simulink model "simulink_02"  (R2023b)
settings: Solver=VariableStepAuto  StartTime=0.0  StopTime=10000  RelTol=1e-3
settings Model: Creator=HP  LastModifiedBy=HP

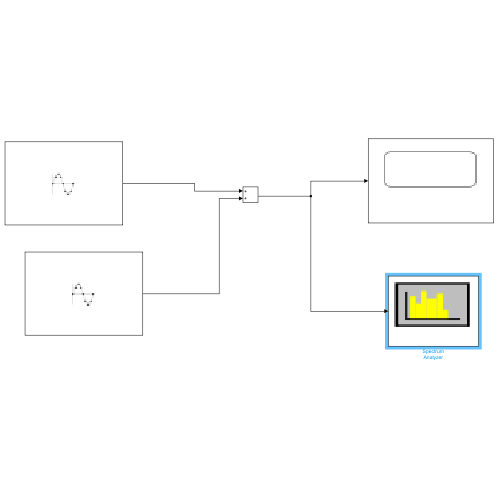
[thumbnail: Simulink's stored preview of the top-level diagram]
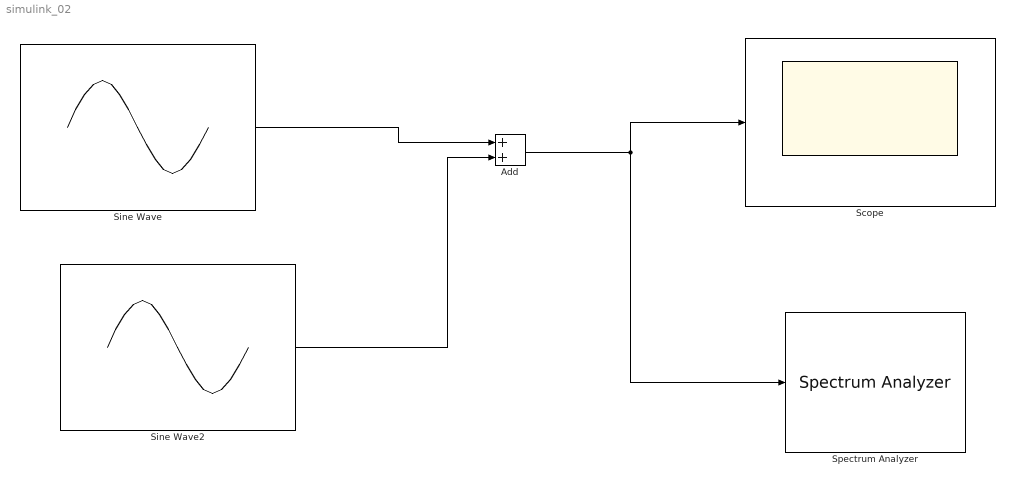
== system simulink_02 ==
  Add : Sum
  Scope : Scope
  Sine Wave : Sin  SineType=Sample based  SampleTime=1
  Sine Wave2 : Sin  SineType=Sample based  SampleTime=1  Offset=5
  Spectrum Analyzer : SpectrumAnalyzer  WindowPosition=[276.000000,58.000000,803.000000,500.000000,]  ScopeFrameLocation=window  Span=1  StartFrequency=-0.5  StopFrequency=0.5  YLimits=[-356.70024064,-288.24939705]
  wires:
  Sine Wave/1 -> Add/1
  Sine Wave2/1 -> Add/2
  Add/1 -> Spectrum Analyzer/1, Scope/1
